simulink model "pump_new_31_03_2023"  (R2020a)
settings: Solver=ode15s  StartTime=0.0  StopTime=0.5  MaxStep=0.0001  RelTol=1e-7  AbsTol=1e-7  EnableMultiTasking=on
libraries: nesl_utility x4, fl_lib x3
settings Model: Creator=123iv  LastModifiedBy=19med
settings SolverCC: AutoScaleAbsTol=off
settings DataIOCC: LimitDataPoints=on  ReturnWorkspaceOutputs=off
settings OptimizationCC: LifeSpan=inf
settings DebuggingCC: AllowSymbolicDim=off  SFUnexpectedBacktrackingDiag=warning  SFNoUnconditionalDefaultTransitionDiag=warning  SFExecutionAtInitializationDiag=none  ArithmeticOperatorsInVariantConditions=warning
settings SFSimCC: SimUseLocalCustomCode=off  CustomCodeUndefinedFunction=UseInterfaceOnly
settings RTWCC: RTWUseLocalCustomCode=off
settings CodeAppCC: StateflowObjectComments=on
settings GRTTargetCC: TargetLangStandard=C89/C90 (ANSI)
settings ConfigComp: CovMetricSettings=dw  CovHtmlReporting=on  CovSaveCumulativeToWorkspaceVar=on  CovSaveSingleToWorkspaceVar=on  CovExternalEMLEnable=off  CovSFcnEnable=off
settings SimscapeCC: SimscapeNormalizeSystem=off  SimscapeLogType=all  SimscapeLogDataHistory=10000

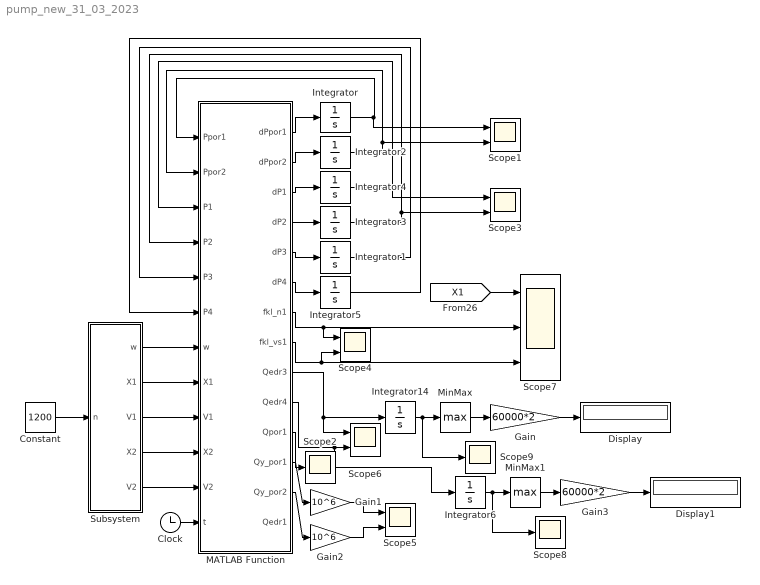
== system pump_new_31_03_2023 ==
  Clock : Clock
  Constant : Constant  Value=1200
  Display : Display
  Display1 : Display
  Gain : Gain  Gain=60000*2
  Gain1 : Gain  Gain=10^6
  Gain2 : Gain  Gain=10^6
  Gain3 : Gain  Gain=60000*2
  Integrator{,1..6,14} (8 alike) : Integrator
  MATLAB Function : MATLAB Function  TreatAsAtomicUnit=on
  MinMax : MinMax  Function=max
  MinMax1 : MinMax  Function=max
  Scope{1,3..6} (5 alike) : Scope  NumInputPorts=2
  Scope2 : Scope
  Scope7 : Scope  NumInputPorts=3
  Scope8 : Scope
  Scope9 : Scope
  Subsystem : Subsystem
  wires:
  MATLAB Function/3(dP1) -> Integrator4/1
  MATLAB Function/1(dPpor1) -> Integrator/1
  MATLAB Function/2(dPpor2) -> Integrator2/1
  Clock/1 -> MATLAB Function/12(t)
  MATLAB Function/5(dP3) -> Integrator1/1
  MATLAB Function/11(Qpor1) -> Scope2/1
  Constant/1 -> Subsystem/1(n)
  Subsystem/1(w) -> MATLAB Function/7(w)
  MATLAB Function/9(Qedr3) -> Integrator14/1, Scope6/1
  MATLAB Function/10(Qedr4) -> Integrator6/1, Scope6/2
  MATLAB Function/7(fkl_n1) -> Scope7/2, Scope4/1
  MATLAB Function/8(fkl_vs1) -> Scope4/2, Scope7/3
  [X1] -> Scope7/1
  Subsystem/2(X1) -> MATLAB Function/8(X1)
  Subsystem/3(V1) -> MATLAB Function/9(V1)
  Gain/1 -> Display/1
  MinMax/1 -> Gain/1
  Integrator14/1 -> Scope9/1, MinMax/1
  MATLAB Function/4(dP2) -> Integrator3/1
  MATLAB Function/6(dP4) -> Integrator5/1
  Integrator/1 -> Scope1/1, MATLAB Function/1(Ppor1)
  Integrator2/1 -> Scope1/2, MATLAB Function/2(Ppor2)
  Integrator4/1 -> MATLAB Function/3(P1), Scope3/1
  Integrator3/1 -> Scope3/2, MATLAB Function/4(P2)
  Integrator1/1 -> MATLAB Function/5(P3)
  Integrator5/1 -> MATLAB Function/6(P4)
  Subsystem/4(X2) -> MATLAB Function/10(X2)
  Subsystem/5(V2) -> MATLAB Function/11(V2)
  Gain1/1 -> Scope5/1
  Gain2/1 -> Scope5/2
  Integrator6/1 -> MinMax1/1, Scope8/1
  MinMax1/1 -> Gain3/1
  Gain3/1 -> Display1/1
  MATLAB Function/12(Qy_por1) -> Gain1/1
  MATLAB Function/13(Qy_por2) -> Gain2/1

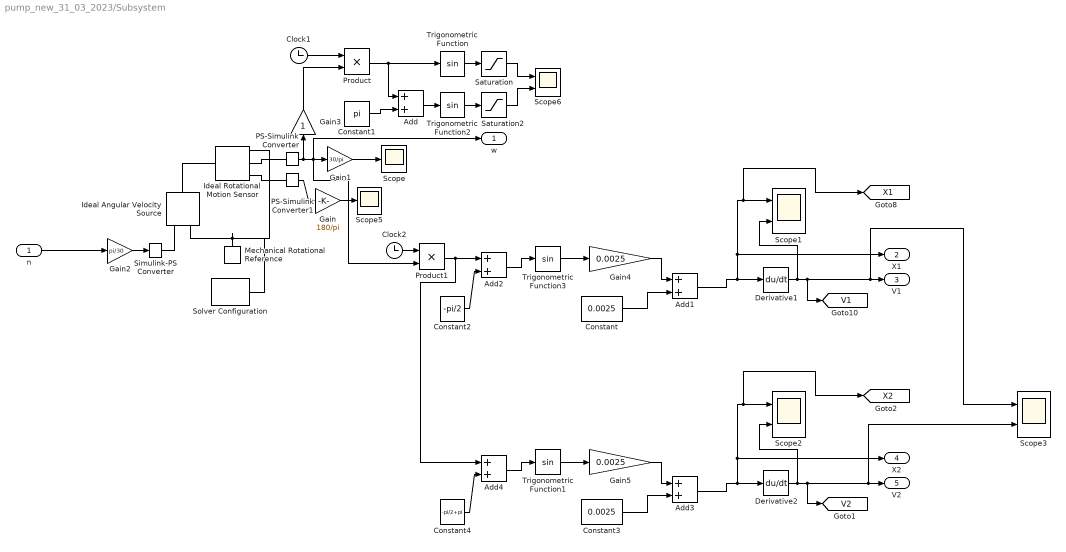
== system pump_new_31_03_2023/Subsystem ==
  n : Inport
  Add{,1..4} (5 alike) : Sum
  Clock1 : Clock
  Clock2 : Clock
  Constant : Constant  Value=0.0025
  Constant1 : Constant  Value=pi
  Constant2 : Constant  Value=-pi/2
  Constant3 : Constant  Value=0.0025
  Constant4 : Constant  Value=-pi/2+pi
  Derivative1 : Derivative
  Derivative2 : Derivative
  Gain : Gain  Gain=180/pi
  Gain1 : Gain  Gain=30/pi
  Gain2 : Gain  Gain=pi/30
  Gain3 : Gain
  Gain4 : Gain  Gain=0.0025
  Gain5 : Gain  Gain=0.0025
  Ideal Angular Velocity Source : fl_lib/Mechanical/Mechanical Sources/Ideal Angular Velocity Source
  Ideal Rotational Motion Sensor : fl_lib/Mechanical/Mechanical Sensors/Ideal Rotational Motion Sensor  wrap_angle=simscape.enum.onoff.on  offset=0 rad
  Mechanical Rotational Reference : fl_lib/Mechanical/Rotational Elements/Mechanical Rotational Reference
  PS-Simulink Converter : nesl_utility/PS-Simulink Converter  PhysicalDomain=network_engine_domain  SubClassName=ps_output  LeftPortType=input  RightPortType=output  PseudoPeriodic=off  Frequencies=[]  Unit=inherit  AffineConversion=off
  PS-Simulink Converter1 : nesl_utility/PS-Simulink Converter  PhysicalDomain=network_engine_domain  SubClassName=ps_output  LeftPortType=input  RightPortType=output  PseudoPeriodic=off  Frequencies=[]  Unit=inherit  AffineConversion=off
  Product : Product
  Product1 : Product
  Saturation : Saturate  UpperLimit=10  LowerLimit=0
  Saturation2 : Saturate  UpperLimit=10  LowerLimit=0
  Scope : Scope
  Scope{1..3,6} (4 alike) : Scope  NumInputPorts=2
  Scope5 : Scope
  Simulink-PS Converter : nesl_utility/Simulink-PS Converter  PhysicalDomain=network_engine_domain  SubClassName=ps_input  LeftPortType=input  RightPortType=output  PseudoPeriodic=off  Frequencies=[]  NoiseDistribution=none  NoiseParameters=[]  Unit=1  AffineConversion=off  FilteringAndDerivatives=provide  SimscapeFilterOrder=1  InputFilterTimeConstant=0.001  UdotUserProvided=0
  Solver Configuration : nesl_utility/Solver Configuration  PhysicalDomain=network_engine_domain  SubClassName=solver  LeftPortType=input  RightPortType=generic  Tones=[]  Harmonics=[]  SimulateNoise=off  Profile=off  UseLocalSampling=off  EnableSwitchedLinearOptims=on  FrequencyDomain=off  UseCCode=off  RelTol=0.001  AbsTol=1e-06  MinStep=1e-09  ToWorkspace=off  RevertToSquareIcSolve=off  NumHomotopyIterations=100  PhasorMode=off  PhasorModeNumHarmonics=1  DoDC=off  ResidualTolerance=1e-09  UseLocalSolver=off  LocalSolverChoice=NE_BACKWARD_EULER_ADVANCER  LocalSolverSampleTime=0.001  DoFixedCost=off  MaxNonlinIter=3  MaxModeIter=2  LinearAlgebra=auto  EquationFormulation=NE_TIME_EF  DelaysMemoryBudget=1024  AutomaticFiltering=on  FilteringTimeConstant=0.001  PartitionStorageMethod=AS_NEEDED  PartitionMemoryBudget=1024  PartitionMethod=ROBUST
  Trigonometric Function{,1..3} (4 alike) : Trigonometry
  w : Outport
  X1 : Outport  Port=2
  V1 : Outport  Port=3
  X2 : Outport  Port=4
  V2 : Outport  Port=5
  tag scope: V1=global, V2=global, X1=global, X2=global
  wires:
  Trigonometric Function/1 -> Saturation/1
  Gain1/1 -> Scope/1
  Gain2/1 -> Simulink-PS Converter/1
  Constant1/1 -> Add/2
  PS-Simulink Converter1/1 -> Gain/1
  Product/1 -> Add/1, Trigonometric Function/1
  Gain3/1 -> Product/2
  Saturation2/1 -> Scope6/2
  Clock1/1 -> Product/1
  Gain/1 -> Scope5/1
  Saturation/1 -> Scope6/1
  n/1 -> Gain2/1
  Add/1 -> Trigonometric Function2/1
  Trigonometric Function2/1 -> Saturation2/1
  Derivative1/1 -> [V1], Scope3/1, V1/1, Scope1/2
  Gain4/1 -> Add1/1
  Trigonometric Function3/1 -> Gain4/1
  Clock2/1 -> Product1/1
  PS-Simulink Converter/1 -> Gain3/1, Product1/2, w/1, Gain1/1
  Add1/1 -> X1/1, [X1], Scope1/1, Derivative1/1
  Constant/1 -> Add1/2
  Add2/1 -> Trigonometric Function3/1
  Constant2/1 -> Add2/2
  Constant4/1 -> Add4/2
  Add4/1 -> Trigonometric Function1/1
  Product1/1 -> Add4/1, Add2/1
  Constant3/1 -> Add3/2
  Add3/1 -> Derivative2/1, Scope2/1, [X2], X2/1
  Trigonometric Function1/1 -> Gain5/1
  Gain5/1 -> Add3/1
  Derivative2/1 -> Scope2/2, Scope3/2, V2/1, [V2]
  connections:
  Mechanical Rotational Reference/LConn1 -- Solver Configuration/RConn1 -- Ideal Rotational Motion Sensor/RConn1 -- Ideal Angular Velocity Source/RConn2
  PS-Simulink Converter/LConn1 -- Ideal Rotational Motion Sensor/RConn2
  PS-Simulink Converter1/LConn1 -- Ideal Rotational Motion Sensor/RConn3
  Simulink-PS Converter/RConn1 -- Ideal Angular Velocity Source/RConn1
  Ideal Rotational Motion Sensor/LConn1 -- Ideal Angular Velocity Source/LConn1

== matlab function pump_new_31_03_2023/MATLAB Function ==
  data: Ppor1 input; Ppor2 input; P1 input; P2 input; dPpor1 output; P3 input; P4 input; w input; dPpor2 output; dP1 output; dP2 output; X1 input; V1 input; X2 input; V2 input; t input; dP3 output; dP4 output; fkl_n1 output; fkl_vs1 output; Qedr3 output; Qedr4 output; Qpor1 output; Qy_por1 output; Qy_por2 output; Qedr1 output
function [dPpor1,dPpor2,dP1,dP2,dP3,dP4,fkl_n1, fkl_vs1,Qedr3,Qedr4,Qpor1, Qy_por1,  Qy_por2, Qedr1] = fcn(Ppor1,Ppor2, P1,P2,P3, P4,w, X1,V1,X2,V2, t)
%ход 5 мм

Ddr=0.005;
Dkl=0.004;%диаметр отверстия клапана
Dpor=13*10^-3; %диаметр поршня
Skl=pi*(Dkl^2)/4;% площадь торца клапана
Spr = (28.19*2.5)*10^-6;% площадь проточки золотника
E=2060000000;
Wn=4*10^-7;
W1 = Wn;
W2 = Wn;
W3 = Wn;
W4 = Wn;

mu = 1003*10^-6;% Па с, коэфф динамической вязкости воды при 20 С
L=30*10^-3; %м, длина поршня, без учета канавок
MUedr=0.7;
MUkl=0.6;
fedr1 = (pi*(Ddr^2)/4);
fedr2 = (pi*(Ddr^2)/4);
fedr3 = (pi*(Ddr^2)/4)/17.5;%35;%70; %%дросель на нагнетании
fedr4 = (pi*(Ddr^2)/4)/1;%2.5;%5;%%дросель на всасывании
Patm=100000;
% Patm=1;
ro=1000;
Spor = (pi*Dpor^2)/4; %площадь поршня
Wpor=10*10^-7;%W0 > (Spor*Xmax=6.63e-07)
%%%
%d=0.0001*10^-3;% зазор между поршнем и гильзой
d=(0.014+0.011)*10^-3;% зазор между поршнем и гильзой
fdry=((pi*((Dpor+d)^2)/4)-Spor);%% площадь утечки поршня

dz = 0.01*10^-3;%  зазор между золотником и обоймой
fdry_zn = (28.19*10^-3)*dz;% площадь утечки золотника
fdry_zvs = (28.19*10^-3)*dz;% площадь утечки золотника
%%%%%%%%% площадь живого сечения клапана 1
fkl_n1 = Spr*sin(w*t);
fkl_vs1 = Spr*sin(w*t+pi);
if (fkl_n1<0) 
    fkl_n1=0;
end
if (fkl_n1>Skl) 
    fkl_n1=Skl;
end
if (fkl_vs1<0) 
    fkl_vs1=0;
end
if (fkl_vs1>Skl) 
    fkl_vs1=Skl;
end
%%%%%%%%%%
%%%%%%%%% площадь живого сечения клапана 2
fkl_n2 = Spr*sin(w*t+pi);
fkl_vs2 = Spr*sin(w*t+2*pi);
if (fkl_n2<0) 
    fkl_n2=0;
end
if (fkl_n2>Skl) 
    fkl_n2=Skl;
end
if (fkl_vs2<0) 
    fkl_vs2=0;
end
if (fkl_vs2>Skl) 
    fkl_vs2=Skl;
end
%%%%%%%%%%

Qedr1=MUedr*fedr1*((2/ro*(abs(Ppor1-P3)))^(1/2))*sign(Ppor1-P3);
Qedr2=MUedr*fedr2*((2/ro*(abs(Ppor2-P4)))^(1/2))*sign(Ppor2-P4);
Qedr3=MUedr*fedr3*((2/ro*(abs(P1-Patm)))^(1/2))*sign(P1-Patm);
Qedr4=MUedr*fedr4*((2/ro*(abs(Patm-P2)))^(1/2))*sign(Patm-P2);

%расход рабочей жидкости при открытии клапана нагнетания 1
Qkl_n1=MUkl*fkl_n1*((2/ro*(abs(P3-P1)))^(1/2))*sign(P3-P1);
%расход рабочей жидкости при открытии клапанавсасывания 1
Qkl_vs1=MUkl*fkl_vs1*((2/ro*(abs(P2-P3)))^(1/2))*sign(P2-P3);
%расход рабочей жидкости при открытии клапана нагнетания 2
Qkl_n2=MUkl*fkl_n2*((2/ro*(abs(P4-P1)))^(1/2))*sign(P4-P1);
%расход рабочей жидкости при открытии клапанавсасывания 2
Qkl_vs2=MUkl*fkl_vs2*((2/ro*(abs(P2-P4)))^(1/2))*sign(P2-P4);


Qpor1=V1*Spor;
Qpor2=V2*Spor;
%%%%утечка поршней
% Qy_por1=MUedr*fdry*((2/ro*(abs(Ppor1-Patm)))^(1/2))*sign(Ppor1-Patm);%утечка поршня1 %зазор 0,01мм
% Qy_por2=MUedr*fdry*((2/ro*(abs(Ppor2-Patm)))^(1/2))*sign(Ppor2-Patm);%утечка поршня2 %зазор 0,01мм
Qy_por1 = pi*(Dpor+d)*((((Ppor1-Patm)*d^3)/(12*mu*L))+(V1*d/2));
Qy_por2 = pi*(Dpor+d)*((((Ppor2-Patm)*d^3)/(12*mu*L))+(V2*d/2));
%%%
% Qy_n=MUdr*fdry_zn*((2/ro*(abs(Pn-P3)))^(1/2))*sign(Pn-P3);%утечка золотника  %зазор 0,01мм
% Qy_vs=MUdr*fdry_zvs*((2/ro*(abs(P3-Pvs)))^(1/2))*sign(P3-Pvs);%утечка золотника  %зазор 0,01мм
Qy_n =0;
Qy_vs = 0;
%%%%%%%%%
%давление в поршневых полостях
dPpor1=(Qpor1-Qedr1-Qy_por1)*E/(Wpor-Spor*X1);
dPpor2=(Qpor2-Qedr2-Qy_por2)*E/(Wpor-Spor*X2);
%
dP1 = (Qkl_n1+Qkl_n2-Qedr3)*E/(W1);
dP2 = (Qedr4-Qkl_vs1-Qkl_vs2)*E/(W2);
dP3 = (Qedr1-Qkl_n1+Qkl_vs1)*E/(W3);
dP4 = (Qedr2-Qkl_n2+Qkl_vs2)*E/(W4);



%%%%%%%%%%%%%%%%
